simulink model "robots"  (Simulink 9.2)
settings: Solver=VariableStepAuto  StartTime=0.0  StopTime=20  MaxStep=1e-3  RelTol=1e-3
settings Model: Creator=jinwooro  LastModifiedBy=jinwooro
settings DataIOCC: LimitDataPoints=off  SaveFormat=Dataset  SignalLoggingSaveFormat=Dataset
settings OptimizationCC: LifeSpan=auto
settings DebuggingCC: UnderspecifiedInitializationDetection=Simplified  MergeDetectMultiDrivingBlocksExec=error  FcnCallInpInsideContextMsg=error  StateNameClashWarn=none  SFUnexpectedBacktrackingDiag=error  SFNoUnconditionalDefaultTransitionDiag=error  SFExecutionAtInitializationDiag=warning
settings HardwareCC: ProdBitPerPointer=64  ProdBitPerSizeT=64  ProdBitPerPtrDiffT=64  ProdLargestAtomicFloat=Float  ProdIntDivRoundTo=Zero  ProdEndianess=LittleEndian  ProdWordSize=64  ProdHWDeviceType=Intel->x86-64 (Windows64)
settings ModelReferenceCC: PropagateSignalLabelsOutOfModel=on
settings SFSimCC: SimUseLocalCustomCode=on
settings RTWCC: RTWUseLocalCustomCode=on
settings CodeAppCC: StateflowObjectComments=off
settings GRTTargetCC: TargetLangStandard=C99 (ISO)  GeneratePreprocessorConditionals=Use local settings  CombineOutputUpdateFcns=on  GRTInterface=off
settings ConfigComp: CovMetricSettings=dwe  CovHtmlReporting=off  CovSaveCumulativeToWorkspaceVar=off  CovSaveSingleToWorkspaceVar=off  CovExternalEMLEnable=on

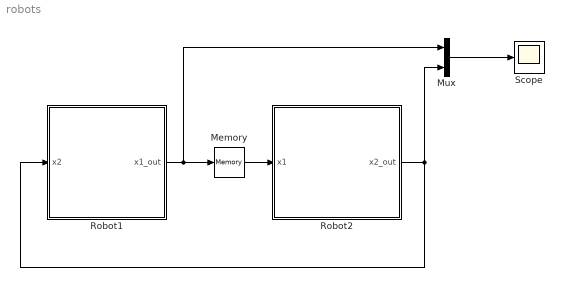
== system robots ==
  Memory : Memory
  Mux : Mux  Inputs=2
  Robot1 : Stateflow chart  TreatAsAtomicUnit=on
  Robot2 : Stateflow chart  TreatAsAtomicUnit=on
  Scope : Scope
  wires:
  Mux/1 -> Scope/1
  Robot1/1(x1_out) -> Memory/1, Mux/1
  Memory/1 -> Robot2/1(x1)
  Robot2/1(x2_out) -> Robot1/1(x2), Mux/2

== stateflow chart Robot2 ==
  settings: updateMethod=CONTINUOUS
  state Approach
    du:
    x2_dot = 0.5 * (20 - x2) + 0.5;
    x2_out = x2;
  state Wait
    du:
    x2_dot = 0;
    x2_out = x2;
  state Transport
    du:
    x2_dot = 2;
    x2_out = x2;
  (default) -> Approach : {
      | x2 = 5;
      | }
  Wait -> Transport : [x1 - x2 >= 0]
  Approach -> Wait : [abs(20- x2) == 0]
  Transport -> Wait : [x2 - x1 >= 0.1]
  data: x2 local double; x2_out output double; x1 input double
  data x2 settings: updateMethod=SF_CONTINUOUS_TIME_DATA

== stateflow chart Robot1 ==
  settings: updateMethod=CONTINUOUS
  state Approach
    du:
    x1_dot = 0.5 * (20 - x1) + 0.3;
    x1_out = x1;
  state Wait
    du:
    x1_dot = 0;
    x1_out = x1;
  state Transport
    du:
    x1_dot = 2;
    x1_out = x1;
  (default) -> Approach : {
      | x1 = 0;
      | }
  Wait -> Transport : [(x2-x1) >= 0]
  Approach -> Wait : [abs(20 - x1) == 0]
  Transport -> Wait : [ x1-x2 >= 0.1 ]
  data: x1 local double; x1_out output double; x2 input double
  data x1 settings: updateMethod=SF_CONTINUOUS_TIME_DATA
